simulink model "mqsls_sim_6dof_ideal"  (R2024b)
settings: configuration reference "prj_default_config" (kept outside this file)
StartFcn:
  | run('control_init.m');
undefined symbols (not defined in the file): force, moment, timestamp
libraries: mqlib x3
settings Model: Creator=yangyu  LastModifiedBy=yangyu
settings ConfigSetRef: SourceName=prj_default_config  SourceLocation=Base Workspace

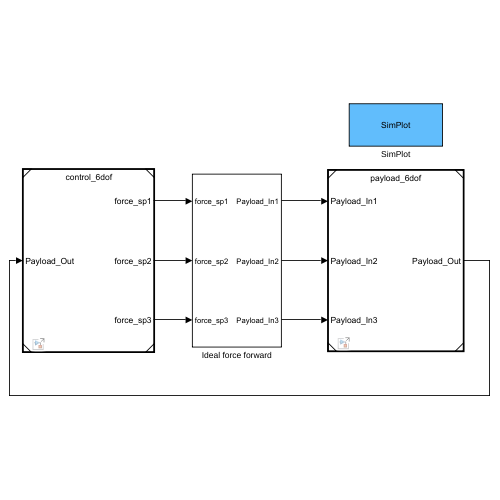
[thumbnail: Simulink's stored preview of the top-level diagram]
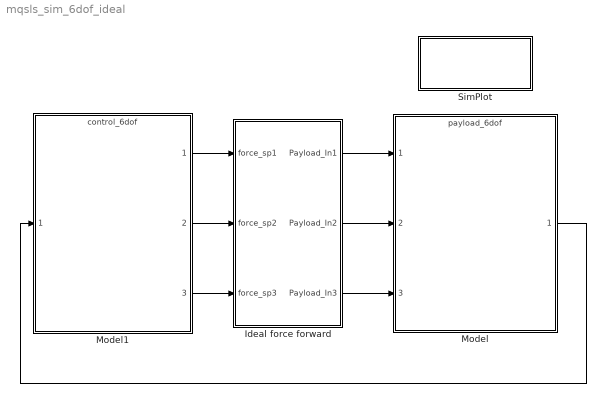
== system mqsls_sim_6dof_ideal ==
  Ideal force forward : Subsystem
  Model : ModelReference  ModelNameDialog=payload_6dof  SimulationMode=Normal  ModelReferenceVersion=1.102
  Model1 : ModelReference  ModelNameDialog=control_6dof  SimulationMode=Normal  ModelReferenceVersion=1.419
  SimPlot : Subsystem
      settings: OpenFcn=run('simplot.m');
      mask Display: disp('SimPlot');
  wires:
  Ideal force forward/3(Payload_In3) -> Model/3
  Ideal force forward/2(Payload_In2) -> Model/2
  Ideal force forward/1(Payload_In1) -> Model/1
  Model/1 -> Model1/1
  Model1/1 -> Ideal force forward/1(force_sp1)
  Model1/2 -> Ideal force forward/2(force_sp2)
  Model1/3 -> Ideal force forward/3(force_sp3)

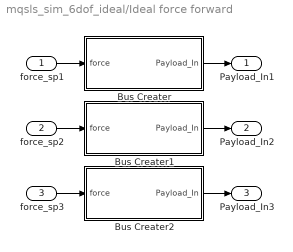
== system mqsls_sim_6dof_ideal/Ideal force forward ==
  force_sp1 : Inport
  force_sp2 : Inport  Port=2
  force_sp3 : Inport  Port=3
  Bus Creater : Subsystem
  Bus Creater1 : Subsystem
  Bus Creater2 : Subsystem
  Payload_In1 : Outport  OutDataTypeStr=Bus: Payload_In_Bus
  Payload_In2 : Outport  Port=2  OutDataTypeStr=Bus: Payload_In_Bus
  Payload_In3 : Outport  Port=3  OutDataTypeStr=Bus: Payload_In_Bus
  wires:
  Bus Creater/1(Payload_In) -> Payload_In1/1
  force_sp3/1 -> Bus Creater2/1(force)
  force_sp1/1 -> Bus Creater/1(force)
  Bus Creater1/1(Payload_In) -> Payload_In2/1
  force_sp2/1 -> Bus Creater1/1(force)
  Bus Creater2/1(Payload_In) -> Payload_In3/1

== system mqsls_sim_6dof_ideal/SimPlot ==

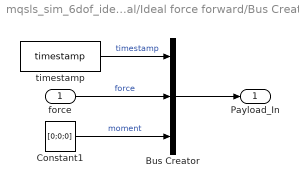
== system mqsls_sim_6dof_ideal/Ideal force forward/Bus Creater ==
  force : Inport
  Bus Creator : BusCreator  Inputs=timestamp,force,moment  OutDataTypeStr=Bus: Payload_In_Bus
  Constant1 : Constant  Value=[0;0;0]  OutDataTypeStr=Inherit: Inherit via back propagation
  timestamp : mqlib/timestamp
  Payload_In : Outport  OutDataTypeStr=Bus: Payload_In_Bus
  wires:
  timestamp/1 -> Bus Creator/1  "timestamp"
  Constant1/1 -> Bus Creator/3  "moment"
  force/1 -> Bus Creator/2  "force"
  Bus Creator/1 -> Payload_In/1

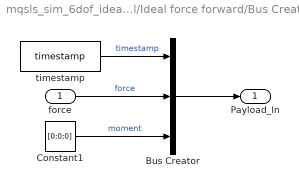
== system mqsls_sim_6dof_ideal/Ideal force forward/Bus Creater1 ==
  force : Inport
  Bus Creator : BusCreator  Inputs=timestamp,force,moment  OutDataTypeStr=Bus: Payload_In_Bus
  Constant1 : Constant  Value=[0;0;0]  OutDataTypeStr=Inherit: Inherit via back propagation
  timestamp : mqlib/timestamp
  Payload_In : Outport  OutDataTypeStr=Bus: Payload_In_Bus
  wires:
  Bus Creator/1 -> Payload_In/1
  force/1 -> Bus Creator/2  "force"
  Constant1/1 -> Bus Creator/3  "moment"
  timestamp/1 -> Bus Creator/1  "timestamp"

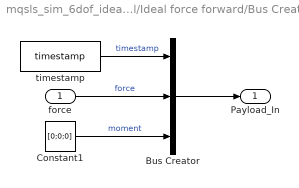
== system mqsls_sim_6dof_ideal/Ideal force forward/Bus Creater2 ==
  force : Inport
  Bus Creator : BusCreator  Inputs=timestamp,force,moment  OutDataTypeStr=Bus: Payload_In_Bus
  Constant1 : Constant  Value=[0;0;0]  OutDataTypeStr=Inherit: Inherit via back propagation
  timestamp : mqlib/timestamp
  Payload_In : Outport  OutDataTypeStr=Bus: Payload_In_Bus
  wires:
  timestamp/1 -> Bus Creator/1  "timestamp"
  Constant1/1 -> Bus Creator/3  "moment"
  force/1 -> Bus Creator/2  "force"
  Bus Creator/1 -> Payload_In/1
